simulink model "task8ss"  (R2017b)
settings: Solver=VariableStepAuto  StartTime=0.0  StopTime=10.0  RelTol=1e-3
values from neighbouring files (symbols this model uses):
  A = [0 1 0 0;(-2*k/m) (-2*c/m) 0 0; 0 0 0 1;0 0 (-2*k*L^2)/J (-2*c*L^2)/J]    [H_inf_ctrl.m]    (also in Task6.m = [0,1,0,0;-ks/ms,-T/ms,ks/ms,0;0,0,0,1;ks/mp,T/mp,-(ks+kp)/mp; Task8.m)
  B = [0 0 0 0;k/m c/m k/m c/m;0 0 0 0;-k*L/J -c*L/J k*L/J c*L/J]    [H_inf_ctrl.m]    (also in Task6.m = [0,0;0,0;0,0;kp/mp,cp/mp]; Task8.m)
  C = [1 0 0 0;0 0 1 0]    [H_inf_ctrl.m]    (also in Task6.m = diag(o); Task8.m)
  D = [0 0 0 0;0 0 0 0]    [H_inf_ctrl.m]    (also in Task6.m = zeros(4,2); Task8.m)
  f = 8    [H_inf_ctrl.m]    (also in Task6.m = 2; Task8.m; task5.m = 0.5)
  src = 1    [H_inf_ctrl.m]    (also in Task3.m = 3; Task6.m = 3; Task8.m)
undefined symbols (not defined in the file or in its folder): sigbuilder_block
settings Model: Creator=Dell  LastModifiedBy=Dell

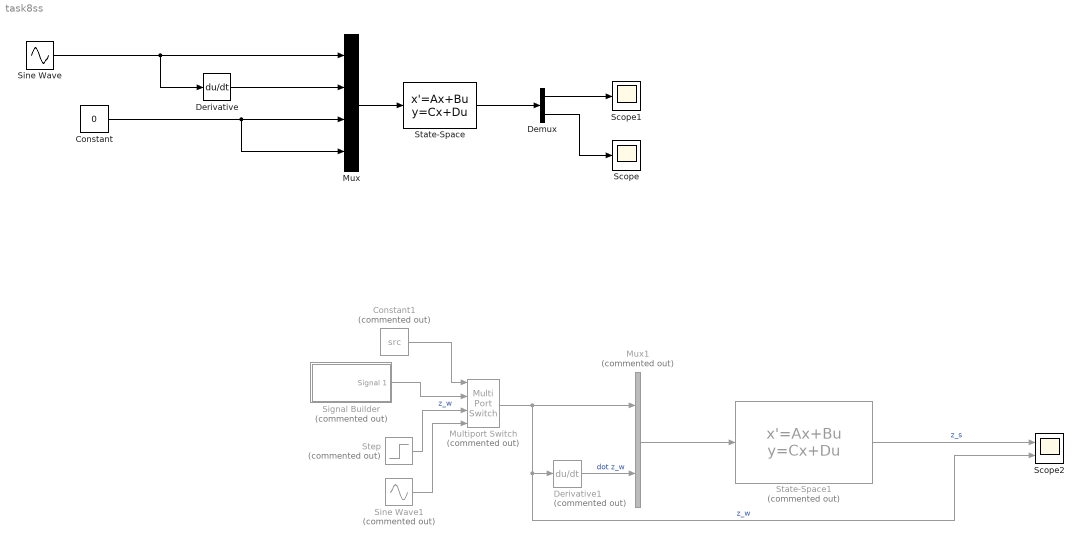
== system task8ss ==
  Constant : Constant  Value=0
  Constant1 : Constant  Commented=on  Value=src
  Demux : Demux  Outputs=2
  Derivative : Derivative
  Derivative1 : Derivative  Commented=on
  Multiport Switch : MultiPortSwitch  Commented=on
  Mux : Mux
  Mux1 : Mux  Commented=on  Inputs=2
  Scope : Scope
  Scope1 : Scope
  Scope2 : Scope  NumInputPorts=2
  Signal Builder : Subsystem  Tag=STV Subsys  Commented=on  LoadFcn=sigbuilder_block('load');  StartFcn=sigbuilder_block('start');  StopFcn=sigbuilder_block('stop');  ClipboardFcn=sigbuilder_block('clipboard');  mask(Sigbuilder block){tuvar=[0:10]}
      mask help: Simulink:masks:SigbuilderBlock_MD
      mask init:
      | if ~strcmp(get_param(bdroot(gcbh),'SimulationStatus'),'stopped') tuvar = sigbuilder_block('maskInit'); end
      settings: CopyFcn=sigbuilder_block('copy');  DeleteFcn=sigbuilder_block('delete');  ModelCloseFcn=sigbuilder_block('modelClose');  PreSaveFcn=sigbuilder_block('preSave');  PauseFcn=sigbuilder_block('pause');  ContinueFcn=sigbuilder_block('continue');  NameChangeFcn=sigbuilder_block('namechange');  OpenFcn=sigbuilder_block('open',[437.6 199.2 550.4 400 ]);  CloseFcn=sigbuilder_block('close');
      mask Display: plot(0, 0, 100, 100,[2, 2, 32, 32, 2], [68, 8, 8, 68, 68],[32, 2], [38, 38], [32, 19, 2],[53, 60, 44], [32, 17, 17, 2],[16, 16, 31, 31]);txt = getActiveGroup(gcbh);text(2, 100, txt,'verticalAlignment', 'top');
  Sine Wave : Sin  Amplitude=0.01  Frequency=2*pi*f  SampleTime=0
  Sine Wave1 : Sin  Commented=on  SampleTime=0
  State-Space : StateSpace  A=A  B=B  C=C  D=D  InitialCondition=0
  State-Space1 : StateSpace  Commented=on  A=A  B=B  C=C  D=D  InitialCondition=0
  Step : Step  Commented=on  After=0.05  SampleTime=0
  wires:
  Mux/1 -> State-Space/1
  Demux/1 -> Scope1/1
  State-Space/1 -> Demux/1
  Demux/2 -> Scope/1
  Sine Wave/1 -> Derivative/1, Mux/1
  Derivative/1 -> Mux/2
  Constant/1 -> Mux/4, Mux/3
  Constant1/1 -> Multiport Switch/1
  Sine Wave1/1 -> Multiport Switch/4
  Signal Builder/1(Signal 1) -> Multiport Switch/2
  Derivative1/1 -> Mux1/2  "dot z_w"
  Step/1 -> Multiport Switch/3  "z_w"
  State-Space1/1 -> Scope2/1  "z_s"
  Mux1/1 -> State-Space1/1
  Multiport Switch/1 -> Mux1/1, Scope2/2, Derivative1/1  "z_w"

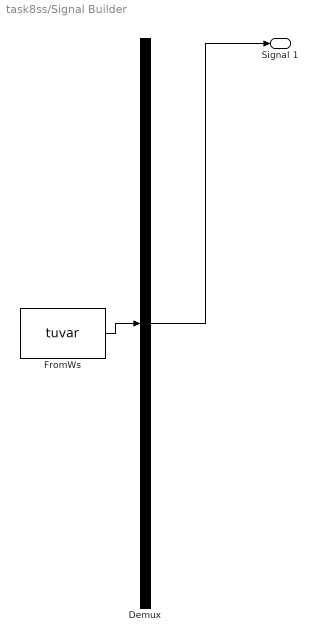
== system task8ss/Signal Builder ==
  Demux : Demux  Tag=STV Demux  Outputs=1
  FromWs : FromWorkspace  Tag=STV FromWs  VariableName=tuvar  SampleTime=0
      SigBuilderData=|
      | common.afterFinalStr = 'Extrapolate'
      | common.sampleTime = 0
      | dataSet.timeRange = [0 10]
      | dataSet.name = 'Group 1'
      | sbobj.Groups.Name = 'Group 1'
      | sbobj.Groups.Signals.Name = 'Signal 1'
      | sbobj.Groups.Signals.XData = [0 4 4 5 5 10]
      | sbobj.Groups.Signals.YData = [0 0 0.05 0.05 0 0]
  Signal 1 : Outport  Tag=STV Outport
  wires:
  Demux/1 -> Signal 1/1
  FromWs/1 -> Demux/1
